simulink model "c2_wideband_filter"  (R2020b)
settings: Solver=FixedStepDiscrete  StartTime=0.0  StopTime=stopTime  FixedStep=2.0833333333333333e-05  RelTol=1e-3
InitFcn:
  | initCallback
StopFcn:
  | stopCallback
values from neighbouring files (symbols this model uses):
  cf = 1000    [modelparameters.m]
undefined symbols (not defined in the file or in its folder): C2coeffs, norm_gainc2
settings Model: Creator=Ross  LastModifiedBy=conno
settings DataIOCC: SaveOutput=off  SaveTime=off  ReturnWorkspaceOutputs=off
settings OptimizationCC: BlockReduction=off  ConditionallyExecuteInputs=off  DefaultParameterBehavior=Inlined
settings DebuggingCC: ReadBeforeWriteMsg=DisableAll  WriteAfterWriteMsg=DisableAll  WriteAfterReadMsg=DisableAll  AlgebraicLoopMsg=error  MultiTaskDSMMsg=none  SingleTaskRateTransMsg=error  PregeneratedLibrarySubsystemCodeDiagnostic=none  ArithmeticOperatorsInVariantConditions=warning
settings HardwareCC: ProdBitPerPointer=32  ProdBitPerSizeT=32  ProdBitPerPtrDiffT=32  ProdLargestAtomicFloat=None  ProdIntDivRoundTo=Undefined  ProdEndianess=Unspecified  ProdWordSize=32  ProdHWDeviceType=ASIC/FPGA->ASIC/FPGA  TargetBitPerPointer=64  TargetBitPerSizeT=64  TargetBitPerPtrDiffT=64  TargetLongLongMode=on  TargetIntDivRoundTo=Zero  TargetEndianess=LittleEndian  TargetWordSize=64  TargetHWDeviceType=Custom Processor->MATLAB Host Computer  ProdEqTarget=off
settings ModelReferenceCC: UpdateModelReferenceTargets=IfOutOfDate
settings SFSimCC: SFSimEcho=off  SimUseLocalCustomCode=off  CustomCodeUndefinedFunction=UseInterfaceOnly
settings RTWCC: RTWUseLocalCustomCode=off

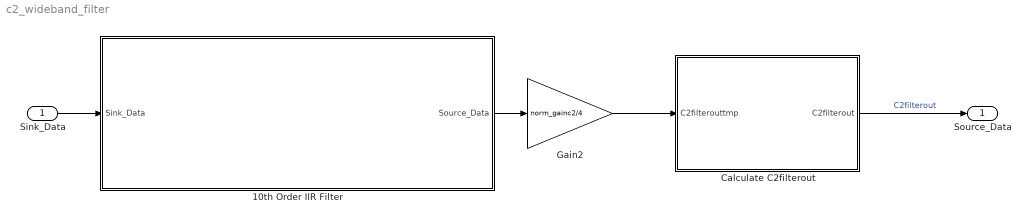
== system c2_wideband_filter ==
  Sink_Data : Inport  OutDataTypeStr=single  PortDimensions=1  SampleTime=[2.0833333333333333e-05,0]
  10th Order IIR Filter : Subsystem
  Calculate C2filterout : Subsystem
  Gain2 : Gain  Gain=norm_gainc2/4
  Source_Data : Outport  OutDataTypeStr=single  PortDimensions=1  SampleTime=[2.0833333333333333e-05,0]  InitialOutput=0  VectorParamsAs1DForOutWhenUnconnected=off
  wires:
  Sink_Data/1 -> 10th Order IIR Filter/1(Sink_Data)
  10th Order IIR Filter/1(Source_Data) -> Gain2/1
  Gain2/1 -> Calculate C2filterout/1(C2filterouttmp)
  Calculate C2filterout/1(C2filterout) -> Source_Data/1  "C2filterout"

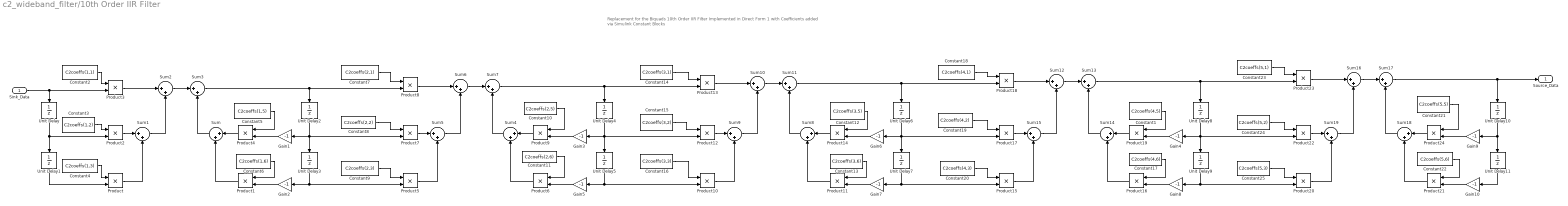
== system c2_wideband_filter/10th Order IIR Filter ==
  note: Replacement for the Biquads
      | 10th Order IIR Filter Implemented in Direct Form 1 with Coefficients added via Simulink Constant Blocks
  Sink_Data : Inport  OutDataTypeStr=single
  Constant1 : Constant  Value=C2coeffs(4,5)  OutDataTypeStr=single  SampleTime=-1
  Constant10 : Constant  Value=C2coeffs(2,5)  OutDataTypeStr=single  SampleTime=-1
  Constant11 : Constant  Value=C2coeffs(2,6)  OutDataTypeStr=single  SampleTime=-1
  Constant12 : Constant  Value=C2coeffs(3,5)  OutDataTypeStr=single  SampleTime=-1
  Constant13 : Constant  Value=C2coeffs(3,6)  OutDataTypeStr=single  SampleTime=-1
  Constant14 : Constant  Value=C2coeffs(3,1)  OutDataTypeStr=single  SampleTime=-1
  Constant15 : Constant  Value=C2coeffs(3,2)  OutDataTypeStr=single  SampleTime=-1
  Constant16 : Constant  Value=C2coeffs(3,3)  OutDataTypeStr=single  SampleTime=-1
  Constant17 : Constant  Value=C2coeffs(4,6)  OutDataTypeStr=single  SampleTime=-1
  Constant18 : Constant  Value=C2coeffs(4,1)  OutDataTypeStr=single  SampleTime=-1
  Constant19 : Constant  Value=C2coeffs(4,2)  OutDataTypeStr=single  SampleTime=-1
  Constant2 : Constant  Value=C2coeffs(1,1)  OutDataTypeStr=single  SampleTime=-1
  Constant20 : Constant  Value=C2coeffs(4,3)  OutDataTypeStr=single  SampleTime=-1
  Constant21 : Constant  Value=C2coeffs(5,5)  OutDataTypeStr=single  SampleTime=-1
  Constant22 : Constant  Value=C2coeffs(5,6)  OutDataTypeStr=single  SampleTime=-1
  Constant23 : Constant  Value=C2coeffs(5,1)  OutDataTypeStr=single  SampleTime=-1
  Constant24 : Constant  Value=C2coeffs(5,2)  OutDataTypeStr=single  SampleTime=-1
  Constant25 : Constant  Value=C2coeffs(5,3)  OutDataTypeStr=single  SampleTime=-1
  Constant3 : Constant  Value=C2coeffs(1,2)  OutDataTypeStr=single  SampleTime=-1
  Constant4 : Constant  Value=C2coeffs(1,3)  OutDataTypeStr=single  SampleTime=-1
  Constant5 : Constant  Value=C2coeffs(1,5)  OutDataTypeStr=single  SampleTime=-1
  Constant6 : Constant  Value=C2coeffs(1,6)  OutDataTypeStr=single  SampleTime=-1
  Constant7 : Constant  Value=C2coeffs(2,1)  OutDataTypeStr=single  SampleTime=-1
  Constant8 : Constant  Value=C2coeffs(2,2)  OutDataTypeStr=single  SampleTime=-1
  Constant9 : Constant  Value=C2coeffs(2,3)  OutDataTypeStr=single  SampleTime=-1
  Gain{1..10} (10 alike) : Gain  Gain=-1
  Product{,1..24} (25 alike) : Product
  Sum{,1..19} (20 alike) : Sum  Inputs=|++
  Unit Delay{,1..11} (12 alike) : UnitDelay  SampleTime=-1  HasFrameUpgradeWarning=on
  Source_Data : Outport  OutDataTypeStr=single
  wires:
  Sum12/1 -> Sum13/1
  Product19/1 -> Sum14/1
  Product1/1 -> Sum/2
  Product24/1 -> Sum18/1
  Constant23/1 -> Product23/1
  Product21/1 -> Sum18/2
  Constant2/1 -> Product3/1
  Constant7/1 -> Product8/1
  Sink_Data/1 -> Unit Delay/1, Product3/2
  Gain8/1 -> Product16/2
  Product8/1 -> Sum6/1
  Constant1/1 -> Product19/1
  Unit Delay4/1 -> Gain3/1, Unit Delay5/1, Product12/2
  Unit Delay9/1 -> Gain8/1, Product20/2
  Product12/1 -> Sum9/1
  Constant20/1 -> Product15/1
  Sum18/1 -> Sum17/2
  Constant24/1 -> Product22/1
  Product11/1 -> Sum8/2
  Unit Delay3/1 -> Gain2/1, Product5/2
  Product15/1 -> Sum15/2
  Product22/1 -> Sum19/1
  Product7/1 -> Sum5/1
  Gain6/1 -> Product14/2
  Product16/1 -> Sum14/2
  Unit Delay5/1 -> Gain5/1, Product10/2
  Sum13/1 -> Product23/2, Unit Delay8/1
  Constant25/1 -> Product20/1
  Constant11/1 -> Product6/1
  Sum7/1 -> Product13/2, Unit Delay4/1
  Unit Delay1/1 -> Product/2
  Product6/1 -> Sum4/2
  Gain7/1 -> Product11/2
  Sum9/1 -> Sum10/2
  Gain1/1 -> Product4/2
  Constant17/1 -> Product16/1
  Sum8/1 -> Sum11/2
  Gain4/1 -> Product19/2
  Sum10/1 -> Sum11/1
  Product14/1 -> Sum8/1
  Gain5/1 -> Product6/2
  Gain9/1 -> Product24/2
  Unit Delay10/1 -> Gain9/1, Unit Delay11/1
  Unit Delay6/1 -> Gain6/1, Unit Delay7/1, Product17/2
  Sum/1 -> Sum3/2
  Sum11/1 -> Product18/2, Unit Delay6/1
  Constant13/1 -> Product11/1
  Product18/1 -> Sum12/1
  Constant15/1 -> Product12/1
  Constant22/1 -> Product21/1
  Sum16/1 -> Sum17/1
  Constant9/1 -> Product5/1
  Constant19/1 -> Product17/1
  Unit Delay7/1 -> Gain7/1, Product15/2
  Unit Delay2/1 -> Gain1/1, Unit Delay3/1, Product7/2
  Constant21/1 -> Product24/1
  Constant3/1 -> Product2/1
  Product20/1 -> Sum19/2
  Product3/1 -> Sum2/1
  Product23/1 -> Sum16/1
  Sum3/1 -> Product8/2, Unit Delay2/1
  Product9/1 -> Sum4/1
  Constant16/1 -> Product10/1
  Sum19/1 -> Sum16/2
  Unit Delay8/1 -> Gain4/1, Unit Delay9/1, Product22/2
  Unit Delay/1 -> Product2/2, Unit Delay1/1
  Gain3/1 -> Product9/2
  Product10/1 -> Sum9/2
  Sum15/1 -> Sum12/2
  Product13/1 -> Sum10/1
  Sum17/1 -> Source_Data/1, Unit Delay10/1
  Gain2/1 -> Product1/2
  Constant14/1 -> Product13/1
  Product17/1 -> Sum15/1
  Product4/1 -> Sum/1
  Constant12/1 -> Product14/1
  Constant18/1 -> Product18/1
  Sum4/1 -> Sum7/2
  Constant4/1 -> Product/1
  Unit Delay11/1 -> Gain10/1
  Constant5/1 -> Product4/1
  Gain10/1 -> Product21/2
  Product2/1 -> Sum1/1
  Product5/1 -> Sum5/2
  Constant10/1 -> Product9/1
  Sum14/1 -> Sum13/2
  Constant8/1 -> Product7/1
  Sum2/1 -> Sum3/1
  Sum6/1 -> Sum7/1
  Sum1/1 -> Sum2/2
  Constant6/1 -> Product1/1
  Product/1 -> Sum1/2
  Sum5/1 -> Sum6/2

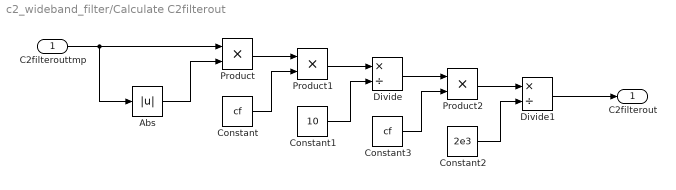
== system c2_wideband_filter/Calculate C2filterout ==
  C2filterouttmp : Inport
  Abs : Abs
  Constant : Constant  Value=cf  OutDataTypeStr=single  SampleTime=-1
  Constant1 : Constant  Value=10  OutDataTypeStr=single  SampleTime=-1
  Constant2 : Constant  Value=2e3  OutDataTypeStr=single  SampleTime=-1
  Constant3 : Constant  Value=cf  OutDataTypeStr=single  SampleTime=-1
  Divide : Product  Inputs=*/  RndMeth=Zero  SaturateOnIntegerOverflow=on
  Divide1 : Product  Inputs=*/  RndMeth=Zero  SaturateOnIntegerOverflow=on
  Product : Product
  Product1 : Product
  Product2 : Product
  C2filterout : Outport  VectorParamsAs1DForOutWhenUnconnected=off
  wires:
  C2filterouttmp/1 -> Product/1, Abs/1
  Abs/1 -> Product/2
  Product/1 -> Product1/1
  Constant/1 -> Product1/2
  Product1/1 -> Divide/1
  Constant1/1 -> Divide/2
  Product2/1 -> Divide1/1
  Constant2/1 -> Divide1/2
  Constant3/1 -> Product2/2
  Divide/1 -> Product2/1
  Divide1/1 -> C2filterout/1
